simulink model "SRM_1DModel"  (R2025a)
settings: Solver=FixedStepAuto  StartTime=0.0  StopTime=.1  FixedStep=1e-5  RelTol=1e-3
InitFcn:
  | %thi =12
  | %thf = 56
  | 
  | %Vdc = 96;
values from neighbouring files (symbols this model uses):
  Nrpm = 1500    [ParamSweep.m]    (also in ParamSweep1D.m = 2500; ParamSweepAndSave.m)
  Vdc = 72    [ParamSweep.m]    (also in ParamSweep1D.m = 96; ParamSweepAndSave.m)
undefined symbols (not defined in the file or in its folder): bp_curr, bp_pos, table_flux
libraries: eeGeneralControl x2, spspowerguiLib x1
settings Model: Creator=PRANJAL  LastModifiedBy=DELL

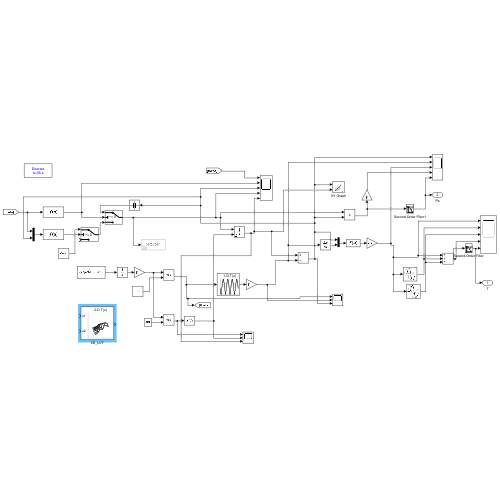
[thumbnail: Simulink's stored preview of the top-level diagram]
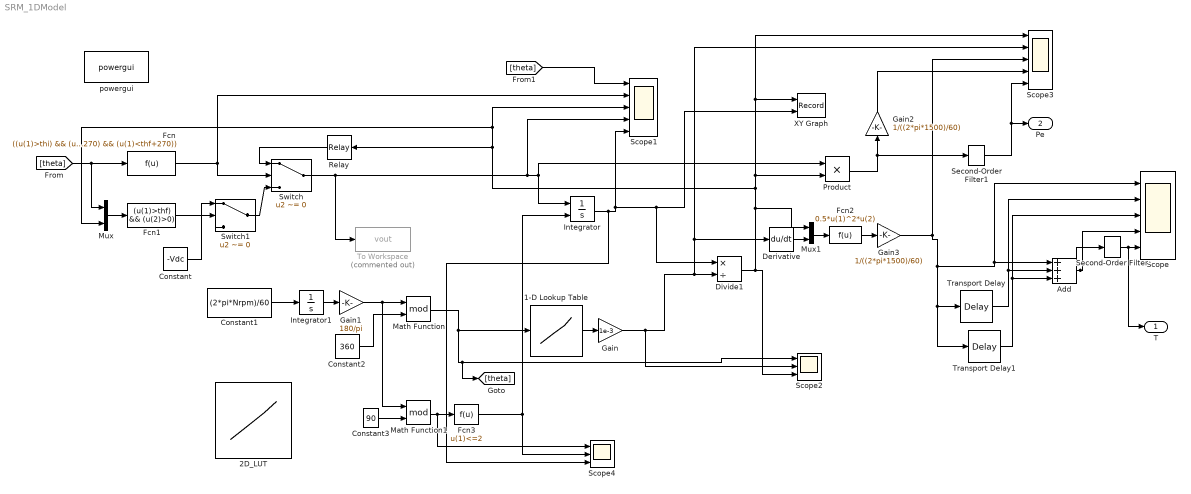
== system SRM_1DModel ==
  1-D Lookup Table : Lookup_n-D  NumberOfTableDimensions=1  BreakpointsForDimension1=[0;1;2;3;4;5;6;7;8;9;10;11;12;13;14;15;16;17;18;19;20;21;22;23;24;25;26;27;28;29;30;31;32;33;34;35;36;37;38;39;40;41;42;43;44;45;46;47;48;49;50;51;52;53;54;55;56;57;58;59;60;61;62;63;64;65;66;67;68;69;70;71;72;73;74;75;76;77;78;79;80;81;82;83;84;85;86;87;88;89;90;91;92;93;94;95;96;97;98;99;100;101;102;103;104;105;106;107;108;109;110;111;112;113;114;115;116;117;118;119;120;121;122;123;124;125;126;127;128;129;130;131;132;133;134;135;136;137;138;139;140;141;142;143;144;145;146;147;148;149;150;151;152;153;154;155;156;157;158;159;160;161;162;163;164;165;166;167;168;169;170;171;172;173;174;175;176;177;178;179;180;181;182;183;184;185;186;187;188;189;190;191;192;193;194;195;196;197;198;199;200;201;202;203;204;205;206;207;208;209;210;211;212;213;214;215;216;217;218;219;220;221;222;223;224;225;226;227;228;229;230;231;232;233;234;235;236;237;238;239;240;241;242;243;244;245;246;247;248;249;250;251;252;253;254;255;256;257;258;259;260;261;262;263;264;265;266;267;268;269;270;271;272;273;274;275;276;277;278;279;280;281;282;283;284;285;286;287;288;289;290;291;292;293;294;295;296;297;298;299;300;301;302;303;304;305;306;307;308;309;310;311;312;313;314;315;316;317;318;319;320;321;322;323;324;325;326;327;328;329;330;331;332;333;334;335;336;337;338;339;340;341;342;343;344;345;346;347;348;349;350;351;352;353;354;355;356;357;358;359;360]  Table=[18.4544;17.70603;16.83468;15.90216;14.98268;14.06655;13.22206;12.21734;11.32744;10.40112;9.625575;9.104048000000001;8.771549;8.561794000000001;8.444464;8.404441;8.443472;8.55996;8.77206;9.105626000000001;9.537259000000001;10.28633;11.32887;12.21728;13.12339;13.8882;14.98626;15.90132;16.75069;17.63253;18.49014;19.38938;20.15801;20.93885;21.69495;22.31111;23.03632;23.71135;24.44817;25.06135;25.66741;26.20106;26.787;27.35776;27.93156;28.45524;29.02524;29.48516;30.06493;30.56454;31.08267;31.62128;32.12755;32.66556;33.19894;33.65025;34.17528;34.63227;34.99652;35.24496;35.29862;35.25616;35.03406;34.68723;34.25277;33.74542;33.26666;32.71355;32.20064;31.63335;31.09965;30.56178;30.06807;29.54679;29.03722;28.45018;27.93047;27.34734;26.79539;26.24744;25.6621;25.05332;24.44143;23.80029;23.13198;22.40847;21.69449;20.97991;20.16516;19.39532;18.4544;17.70603;16.83468;15.90216;14.98268;14.06655;13.22206;12.21734;11.32744;10.40112;9.625575;9.104048000000001;8.771549;8.561794000000001;8.444464;8.404441;8.443472;8.55996;8.77206;9.105626000000001;9.537259000000001;10.28633;11.32887;12.21728;13.12339;13.8882;14.98626;15.90132;16.75069;17.63253;18.49014;19.38938;20.15801;20.93885;21.69495;22.31111;23.03632;23.71135;24.44817;25.06135;25.66741;26.20106;26.787;27.35776;27.93156;28.45524;29.02524;29.48516;30.06493;30.56454;31.08267;31.62128;32.12755;32.66556;33.19894;33.65025;34.17528;34.63227;34.99652;35.24496;35.29862;35.25616;35.03406;34.68723;34.25277;33.74542;33.26666;32.71355;32.20064;31.63335;31.09965;30.56178;30.06807;29.54679;29.03722;28.45018;27.93047;27.34734;26.79539;26.24744;25.6621;25.05332;24.44143;23.80029;23.13198;22.40847;21.69449;20.97991;20.16516;19.39532;18.4544;17.70603;16.83468;15.90216;14.98268;14.06655;13.22206;12.21734;11.32744;10.40112;9.625575;9.104048000000001;8.771549;8.561794000000001;8.444464;8.404441;8.443472;8.55996;8.77206;9.105626000000001;9.537259000000001;10.28633;11.32887;12.21728;13.12339;13.8882;14.98626;15.90132;16.75069;17.63253;18.49014;19.38938;20.15801;20.93885;21.69495;22.31111;23.03632;23.71135;24.44817;25.06135;25.66741;26.20106;26.787;27.35776;27.93156;28.45524;29.02524;29.48516;30.06493;30.56454;31.08267;31.62128;32.12755;32.66556;33.19894;33.65025;34.17528;34.63227;34.99652;35.24496;35.29862;35.25616;35.03406;34.68723;34.25277;33.74542;33.26666;32.71355;32.20064;31.63335;31.09965;30.56178;30.06807;29.54679;29.03722;28.45018;27.93047;27.34734;26.79539;26.24744;25.6621;25.05332;24.44143;23.80029;23.13198;22.40847;21.69449;20.97991;20.16516;19.39532;18.4544;17.70603;16.83468;15.90216;14.98268;14.06655;13.22206;12.21734;11.32744;10.40112;9.625575;9.104048000000001;8.771549;8.561794000000001;8.444464;8.404441;8.443472;8.55996;8.77206;9.105626000000001;9.537259000000001;10.28633;11.32887;12.21728;13.12339;13.8882;14.98626;15.90132;16.75069;17.63253;18.49014;19.38938;20.15801;20.93885;21.69495;22.31111;23.03632;23.71135;24.44817;25.06135;25.66741;26.20106;26.787;27.35776;27.93156;28.45524;29.02524;29.48516;30.06493;30.56454;31.08267;31.62128;32.12755;32.66556;33.19894;33.65025;34.17528;34.63227;34.99652;35.24496;35.29862;35.25616;35.03406;34.68723;34.25277;33.74542;33.26666;32.71355;32.20064;31.63335;31.09965;30.56178;30.06807;29.54679;29.03722;28.45018;27.93047;27.34734;26.79539;26.24744;25.6621;25.05332;24.44143;23.80029;23.13198;22.40847;21.69449;20.97991;20.16516;19.39532;18.4544]  InternalRulePriority=Speed  RndMeth=Simplest
  2D_LUT : Lookup_n-D  BreakpointsForDimension1=bp_curr  BreakpointsForDimension2=bp_pos  Table=table_flux  InterpMethod=Cubic spline  ExtrapMethod=Cubic spline  InternalRulePriority=Speed  RndMeth=Simplest
      settings: InputPortMap=u0,u1
  Add : Sum  Inputs=+++
  Constant : Constant  Value=-Vdc
  Constant1 : Constant  Value=(2*pi*Nrpm)/60
  Constant2 : Constant  Value=360
  Constant3 : Constant  Value=90
  Derivative : Derivative
  Divide1 : Product  Inputs=*/
  Fcn : Fcn  Expr=((u(1)>thi) && (u(1)<thf)) || ((u(1)>thi+90) && (u(1)<thf+90)) || ((u(1)>thi+180) && (u(1)<thf+180)) || ((u(1)>thi+270) && (u(1)<thf+270))
  Fcn1 : Fcn  Expr=(u(1)>thf) && (u(2)>0)
  Fcn2 : Fcn  Expr=0.5*u(1)^2*u(2)
  Fcn3 : Fcn  Expr=u(1)<=2
  Gain : Gain  Gain=1e-3
  Gain1 : Gain  Gain=180/pi
  Gain2 : Gain  Gain=1/((2*pi*1500)/60)
  Gain3 : Gain  Gain=1/((2*pi*1500)/60)
  Integrator : Integrator  ExternalReset=rising
  Integrator1 : Integrator
  Math Function : Math  Operator=mod
  Math Function1 : Math  Operator=mod
  Mux : Mux  Inputs=2
  Mux1 : Mux  Inputs=2
  Product : Product
  Relay : Relay  OnSwitchValue=10.5  OffSwitchValue=9.5  OnOutputValue=-Vdc  OffOutputValue=Vdc
  Scope : Scope  NumInputPorts=5
      settings: ActiveDisplayYMinimum=-0.90237329382399079  ActiveDisplayYMaximum=4.8000848165919408
  Scope1 : Scope  NumInputPorts=5
      settings: ActiveDisplayYMinimum=-44.9999999999977  ActiveDisplayYMaximum=404.99999999997937  DataLoggingVariableName=ScopeData3
  Scope2 : Scope  NumInputPorts=3
      settings: ActiveDisplayYMinimum=-44.999999999998181  ActiveDisplayYMaximum=404.99999999998369
  Scope3 : Scope  NumInputPorts=5
      settings: ActiveDisplayYMinimum=-1.3967291452123636  ActiveDisplayYMaximum=11.841759422368625  DataLoggingVariableName=ScopeData2
  Scope4 : Scope  NumInputPorts=3
      settings: ActiveDisplayYMinimum=-0.20149768394247602  ActiveDisplayYMaximum=0.60190176977987209  DataLoggingVariableName=ScopeData4
  Second-Order Filter : eeGeneralControl/Second-Order Filter  FilterType=Low-pass  fn=20  Zeta=0.707  Ts=-1  A0=0  Ph0=0  f0=0  b0=0
      settings: LibrarySourceBlock=ee_sl_lib/General Control/Second-Order Filter
  Second-Order Filter1 : eeGeneralControl/Second-Order Filter  FilterType=Low-pass  fn=20  Zeta=0.707  Ts=-1  A0=0  Ph0=0  f0=0  b0=0
      settings: LibrarySourceBlock=ee_sl_lib/General Control/Second-Order Filter
  Switch : Switch  Criteria=u2 ~= 0  Threshold=15  SaturateOnIntegerOverflow=off  InputSameDT=off
  Switch1 : Switch  Criteria=u2 ~= 0  Threshold=15  SaturateOnIntegerOverflow=off  InputSameDT=off
  To Workspace : ToWorkspace  Commented=on  VariableName=vout  SampleTime=-1
  Transport Delay : TransportDelay  DelayTime=1/150  BufferSize=3072
  Transport Delay1 : TransportDelay  DelayTime=2/150  BufferSize=3072
  XY Graph : Record  NumPorts=2.0  FileSettingsInternal="{\"entries\":[{\"content\":{\"excelSettings\":{\"content\":{},\"type\":\"Streamout.ExcelSettings\"},\"parquetSettings\":{\"content\":{},\"type\":\"Streamout.ParquetSettings\"}},\"type\":\"Streamout.FileSettingStorage\",\"uuid\":\"\"}],\"packageUris\":[\"http:\\/\\/schema.mathworks.com\\/mf0\\/streamout_blocks\\/R2020a\"],\"version\":\"1.0\"}"  FrameSettings=[0, 0]  Layout=[1 1]  SignalsInternal="{\"entries\":[{\"content\":{\"signals\":[{\"content\":{\"blockPath\":[],\"dimensions\":[1],\"domain\":\"\",\"lineColor\":\"#a2142f\",\"plots\":[ 1 ],\"port\":1,\"sid\":[\"\"],\"signalID\":1,\"signalName\":\"Divide1\"},\"type\":\"RecordBlkView.Signal\",\"uuid\":\"\"},{\"content\":{\"blockPath\":[],\"dimensions\":[1],\"domain\":\"\",\"lineColor\":\"#139fff\",\"plots\":[ 1 ],\"port\":2,\"sid\":[\"\"],\"signalID\":2,\"signalName\":\"Integrator\"},\"type\":\"RecordBlkView.Signal\",\"uuid\":\"\"}]},\"type\":\"RecordBlkView.InputSignals\",\"uuid\":\"\"}],\"packageUris\":[\"http:\\/\\/schema.mathworks.com\\/mf0\\/streamout_blocks\\/R2020a\"],\"version\":\"1.0\"}"  VisualizationBindings="{\"xyplotplugin\":{\"info\":[{\"series\":[{\"bindingParametersList\":[{\"parameter\":\"X-Axis\",\"signalID\":1,\"signalName\":\"Divide1\"},{\"parameter\":\"Y-Axis\",\"signalID\":2,\"signalName\":\"Integrator\"}],\"seriesID\":0}],\"subplotID\":1}]}}"  CompatibilityTag=XY
  powergui : spspowerguiLib/powergui  Priority=1  SimulationMode=Discrete  SampleTime=10e-6  frequency=60  Iterations=50  frequencyindice=60  Pbase=100e6  ErrMax=1e-4  UnitsV=kV  UnitsW=MW  buscounter=0  FunctionMessages=off  echomessages=off  EnableUseOfTLC=off  CurrentSourceSwitches=off  DisableSnubberDevices=off  DisableRonSwitches=off  DisableVfSwitches=off  DisplayEquations=off  AutomaticDiscreteSolvers=off  SolverType=Tustin/Backward Euler (TBE)  Interpol=off  ExternalGateDelay=off  methode=off  Ts=100  x0status=blocks  SPID=on  SwTol=0  HookPort=off  NonlinearTolerance=1e-4  nMaxIteration=100  ContinueOnMaxIteration=off  RestoreLinks=warning  ResistiveCurrentMeasurement=off  Frange=[0:2:500]  Ylog=off  Xlog=on  ShowGrid=off  save=off  variable=ZData  structure=0  ZoomFFT=off  StartTime=0.0  cycles=1  DisplayStyle=1  fundamental=60  FreqAxis=off  MaxFrequency=1000  frequencyindicesteady=1  RmsSteady=1  display=off
  T : Outport
  Pe : Outport  Port=2
  wires:
  Integrator/1 -> Scope4/3, Scope1/5, XY Graph/2, Divide1/1
  1-D Lookup Table/1 -> Gain/1
  Fcn2/1 -> Gain3/1
  Add/1 -> Scope/4, Second-Order Filter/1
  Constant1/1 -> Integrator1/1
  Gain/1 -> Scope2/2, Scope3/2, Derivative/1, Divide1/2
  Integrator1/1 -> Gain1/1
  Gain1/1 -> Math Function1/1, Math Function/1
  Constant2/1 -> Math Function/2
  Math Function/1 -> [theta], Scope2/1, 1-D Lookup Table/1
  Transport Delay/1 -> Scope/2, Add/2
  Transport Delay1/1 -> Scope/3, Add/3
  Switch/1 -> Scope1/4, Integrator/1, Product/1, To Workspace/1
  Fcn/1 -> Scope1/2, Switch/2
  Relay/1 -> Switch/1
  [theta] -> Mux/1, Fcn/1
  Mux/1 -> Fcn1/1
  Fcn1/1 -> Switch1/2
  Switch1/1 -> Switch/3
  Constant/1 -> Switch1/1
  Mux1/1 -> Fcn2/1
  Divide1/1 -> XY Graph/1, Scope3/1, Product/2, Scope1/3, Mux/2, Relay/1, Mux1/1, Scope2/3
  Derivative/1 -> Mux1/2
  Product/1 -> Gain2/1, Second-Order Filter1/1
  Gain2/1 -> Scope3/4
  Gain3/1 -> Scope3/3, Transport Delay/1, Transport Delay1/1, Scope/1, Add/1
  [theta] -> Scope1/1
  Second-Order Filter/1 -> T/1, Scope/5
  Second-Order Filter1/1 -> Scope3/5, Pe/1
  Constant3/1 -> Math Function1/2
  Math Function1/1 -> Scope4/1, Fcn3/1
  Fcn3/1 -> Scope4/2, Integrator/2
